simulink model "gm_minutiaeextraction_21821"  (R2018b)
settings: Solver=FixedStepDiscrete  StartTime=0.0  StopTime=10  RelTol=1e-3
undefined symbols (not defined in the file or in its folder): gray
libraries: hdlsllib x4, visionsources x1, dspmtrx3 x1
(part 1 of 7)
settings Model: Creator=Administrator  LastModifiedBy=Administrator
settings OptimizationCC: BlockReduction=off  ConditionallyExecuteInputs=off  DefaultParameterBehavior=Inlined
settings DebuggingCC: AlgebraicLoopMsg=error  InheritedTsInSrcMsg=none  SingleTaskRateTransMsg=error
settings HardwareCC: ProdBitPerPointer=32  ProdBitPerSizeT=32  ProdBitPerPtrDiffT=32  ProdLargestAtomicFloat=None  ProdIntDivRoundTo=Undefined  ProdEndianess=Unspecified  ProdWordSize=32  ProdHWDeviceType=ASIC/FPGA->ASIC/FPGA  TargetBitPerPointer=64  TargetBitPerSizeT=64  TargetBitPerPtrDiffT=64  TargetLongLongMode=on  TargetIntDivRoundTo=Zero  TargetEndianess=LittleEndian  TargetWordSize=64  TargetHWDeviceType=Custom Processor->MATLAB Host Computer  ProdEqTarget=off

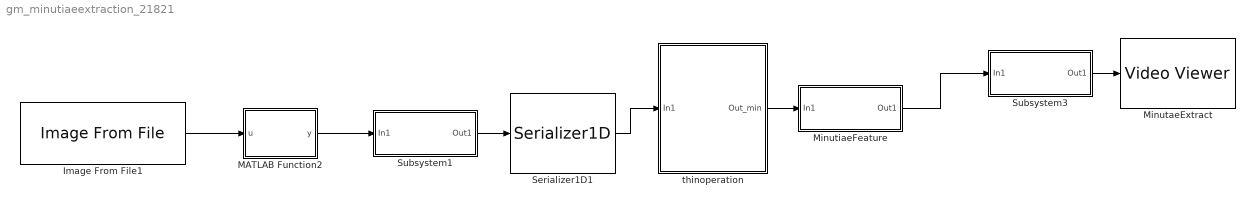
== system gm_minutiaeextraction_21821 ==
  Image From File1 : visionsources/Image From File  Tag=vipblks_nd  FileName=C:\Users\Administrator\Desktop\chapter\thinning\fp1.bmp  imagePorts=One multidimensional signal  Ts=0.1  ImageDataType=uint8  Signed=on  WordLength=16  sdImageDataType=uint(8)  FractionLengthMode=User-defined  FractionLength=15  OutPortLabels=R|G|B
      settings: SourceProductName=Computer Vision System Toolbox
  MATLAB Function2 : MATLAB Function  TreatAsAtomicUnit=on
  MinutaeExtract : VideoViewer  colormapValue=gray(256)  FigPos=[367 903 376 593]
  MinutiaeFeature : Subsystem  TreatAsAtomicUnit=on
  Serializer1D1 : hdlsllib/HDL Operations/Serializer1D  Ratio=1  IdleCycles=0  validIn=off  startOut=off  validOut=off  inputDataDimensions=8192  inputSampleTime=-1  inputSignalType=auto
      settings: SourceProductName=HDL Coder  SourceProductBaseCode=HD
  Subsystem1 : Subsystem
  Subsystem3 : Subsystem
  thinoperation : Subsystem  TreatAsAtomicUnit=on
  wires:
  MinutiaeFeature/1(Out1) -> Subsystem3/1(In1)
  thinoperation/1(Out_min) -> MinutiaeFeature/1(In1)
  Subsystem1/1(Out1) -> Serializer1D1/1
  Image From File1/1 -> MATLAB Function2/1(u)
  MATLAB Function2/1(y) -> Subsystem1/1(In1)
  Serializer1D1/1 -> thinoperation/1(In1)
  Subsystem3/1(Out1) -> MinutaeExtract/1
